simulink model "correlator_core"  (Simulink 7.1)
settings: Solver=ode45  StartTime=0.0  StopTime=10000  RelTol=1e-3
libraries: xbsIndex_r4 x658, cfa_library x168, casper_library_delays x4, casper_library_misc x2
(part 1 of 9)
settings Model: Creator=Administrator  LastModifiedBy=Rurik A Primiani

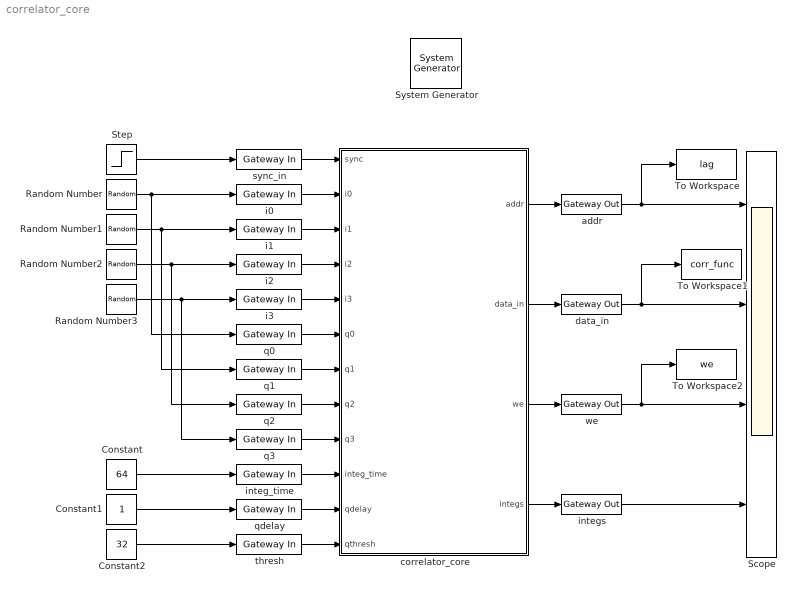
== system correlator_core ==
  " System Generator" : xbsIndex_r4/ System Generator  Tag=genX  SystemSampleTime=-1  xilinxfamily=virtex2p  part=xc2vp50  speed=-7  package=ff1152  synthesis_tool=XST  clock_wrapper=Clock Enables  directory=./correlator_core  testbench=off  simulink_period=1  sysclk_period=100  dcm_input_clock_period=100  incr_netlist=off  trim_vbits=Everywhere in SubSystem  dbl_ovrd=According to Block Masks  core_generation=According to Block Masks  run_coregen=off  deprecated_control=off  eval_field=0  block_type=sysgen
      settings: block_version=10.1.3
  Constant : Constant  Value=64  OutDataType=sfix(16)  OutScaling=2^0
  Constant1 : Constant  OutDataType=sfix(16)  OutScaling=2^0
  Constant2 : Constant  Value=32  OutDataType=sfix(16)  OutScaling=2^0
  Random Number{,1..3} (4 alike) : RandomNumber  Variance=128  Seed=ceil(1000*rand())  SampleTime=0
  Scope : Scope  NumInputPorts=4
      settings: YMin=0~-5e+006~-5~-5  YMax=32.5~5e+007~5~5
  Step : Step  Time=100  SampleTime=0
  To Workspace : ToWorkspace  VariableName=lag  SampleTime=-1  SaveFormat=Array
  To Workspace1 : ToWorkspace  VariableName=corr_func  SampleTime=-1  SaveFormat=Array
  To Workspace2 : ToWorkspace  VariableName=we  SampleTime=-1  SaveFormat=Array
  addr : xbsIndex_r4/Gateway Out  hdl_port=on  timing_constraint=None  locs_specified=off  LOCs={}  block_type=gatewayout
      settings: infoedit="Gateway out block.  Converts Xilinx fixed point inputs into ouputs of type Simulink integer, double, or fixed point.<P><P>Hardware notes:  In hardware these blocks become top level output ports or are discarded, depending on how they are configured."  block_version=10.1.3
  correlator_core : Subsystem
  data_in : xbsIndex_r4/Gateway Out  hdl_port=on  timing_constraint=None  locs_specified=off  LOCs={}  block_type=gatewayout
      settings: infoedit="Gateway out block.  Converts Xilinx fixed point inputs into ouputs of type Simulink integer, double, or fixed point.<P><P>Hardware notes:  In hardware these blocks become top level output ports or are discarded, depending on how they are configured."  block_version=10.1.3
  i{0..3} (4 alike) : xbsIndex_r4/Gateway In  arith_type="Signed  (2's comp)"  n_bits=8  bin_pt=7  quantization=Truncate  overflow=Wrap  period=1  dbl_ovrd=off  timing_constraint=None  locs_specified=off  LOCs={}  block_type=gatewayin
      settings: infoedit="Gateway in block.  Converts inputs of type Simulink integer, double and fixed point to  Xilinx fixed point type.<P><P>Hardware notes:  In hardware these blocks become top level input ports."  block_version=10.1.3
  integ_time : xbsIndex_r4/Gateway In  arith_type=Unsigned  n_bits=32  bin_pt=0  quantization=Truncate  overflow=Wrap  period=1  dbl_ovrd=off  timing_constraint=None  locs_specified=off  LOCs={}  block_type=gatewayin
      settings: infoedit="Gateway in block.  Converts inputs of type Simulink integer, double and fixed point to  Xilinx fixed point type.<P><P>Hardware notes:  In hardware these blocks become top level input ports."  block_version=10.1.3
  integs : xbsIndex_r4/Gateway Out  hdl_port=on  timing_constraint=None  locs_specified=off  LOCs={}  block_type=gatewayout
      settings: infoedit="Gateway out block.  Converts Xilinx fixed point inputs into ouputs of type Simulink integer, double, or fixed point.<P><P>Hardware notes:  In hardware these blocks become top level output ports or are discarded, depending on how they are configured."  block_version=10.1.3
  q{0..3} (4 alike) : xbsIndex_r4/Gateway In  arith_type="Signed  (2's comp)"  n_bits=8  bin_pt=7  quantization=Truncate  overflow=Wrap  period=1  dbl_ovrd=off  timing_constraint=None  locs_specified=off  LOCs={}  block_type=gatewayin
      settings: infoedit="Gateway in block.  Converts inputs of type Simulink integer, double and fixed point to  Xilinx fixed point type.<P><P>Hardware notes:  In hardware these blocks become top level input ports."  block_version=10.1.3
  qdelay : xbsIndex_r4/Gateway In  arith_type=Unsigned  n_bits=11  bin_pt=0  quantization=Truncate  overflow=Wrap  period=1  dbl_ovrd=off  timing_constraint=None  locs_specified=off  LOCs={}  block_type=gatewayin
      settings: infoedit="Gateway in block.  Converts inputs of type Simulink integer, double and fixed point to  Xilinx fixed point type.<P><P>Hardware notes:  In hardware these blocks become top level input ports."  block_version=10.1.3
  sync_in : xbsIndex_r4/Gateway In  arith_type=Boolean  n_bits=16  bin_pt=14  quantization="Round  (unbiased: +/- Inf)"  overflow=Saturate  period=1  dbl_ovrd=off  timing_constraint=None  locs_specified=off  LOCs={}  block_type=gatewayin
      settings: infoedit="Gateway in block.  Converts inputs of type Simulink integer, double and fixed point to  Xilinx fixed point type.<P><P>Hardware notes:  In hardware these blocks become top level input ports."  block_version=10.1.3
  thresh : xbsIndex_r4/Gateway In  arith_type=Unsigned  n_bits=7  bin_pt=0  quantization=Truncate  overflow=Wrap  period=1  dbl_ovrd=off  timing_constraint=None  locs_specified=off  LOCs={}  block_type=gatewayin
      settings: infoedit="Gateway in block.  Converts inputs of type Simulink integer, double and fixed point to  Xilinx fixed point type.<P><P>Hardware notes:  In hardware these blocks become top level input ports."  block_version=10.1.3
  we : xbsIndex_r4/Gateway Out  hdl_port=on  timing_constraint=None  locs_specified=off  LOCs={}  block_type=gatewayout
      settings: infoedit="Gateway out block.  Converts Xilinx fixed point inputs into ouputs of type Simulink integer, double, or fixed point.<P><P>Hardware notes:  In hardware these blocks become top level output ports or are discarded, depending on how they are configured."  block_version=10.1.3
  wires:
  sync_in/1 -> correlator_core/1(sync)
  i0/1 -> correlator_core/2(i0)
  i1/1 -> correlator_core/3(i1)
  i2/1 -> correlator_core/4(i2)
  i3/1 -> correlator_core/5(i3)
  q0/1 -> correlator_core/6(q0)
  q1/1 -> correlator_core/7(q1)
  q2/1 -> correlator_core/8(q2)
  q3/1 -> correlator_core/9(q3)
  correlator_core/1(addr) -> addr/1
  correlator_core/2(data_in) -> data_in/1
  correlator_core/3(we) -> we/1
  Random Number/1 -> i0/1, q0/1
  Random Number1/1 -> i1/1, q1/1
  Random Number2/1 -> i2/1, q2/1
  Random Number3/1 -> i3/1, q3/1
  Step/1 -> sync_in/1
  correlator_core/4(integs) -> integs/1
  integ_time/1 -> correlator_core/10(integ_time)
  Constant/1 -> integ_time/1
  addr/1 -> Scope/1, To Workspace/1
  data_in/1 -> Scope/2, To Workspace1/1
  we/1 -> Scope/3, To Workspace2/1
  integs/1 -> Scope/4
  Constant1/1 -> qdelay/1
  qdelay/1 -> correlator_core/11(qdelay)
  thresh/1 -> correlator_core/12(qthresh)
  Constant2/1 -> thresh/1

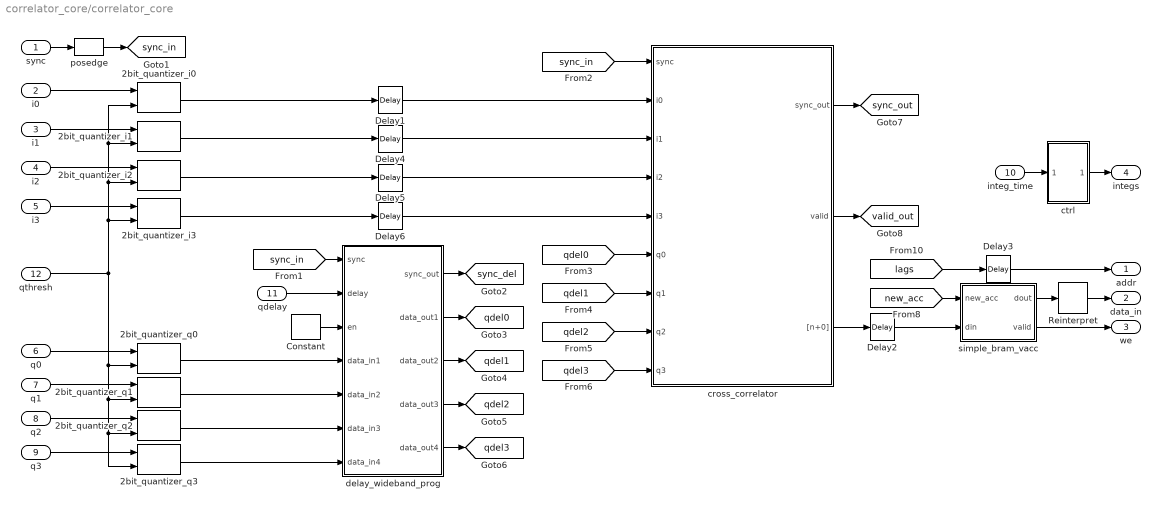
== system correlator_core/correlator_core ==
  sync : Inport
  i0 : Inport  Port=2
  i1 : Inport  Port=3
  i2 : Inport  Port=4
  i3 : Inport  Port=5
  q0 : Inport  Port=6
  q1 : Inport  Port=7
  q2 : Inport  Port=8
  q3 : Inport  Port=9
  integ_time : Inport  Port=10
  qdelay : Inport  Port=11
  qthresh : Inport  Port=12
  2bit_quantizer_i{0..3} (4 alike) : cfa_library/2bit_quantizer  SystemSampleTime=-1  relational_delay=3
  2bit_quantizer_q{0..3} (4 alike) : cfa_library/2bit_quantizer  SystemSampleTime=-1  relational_delay=3
  Constant : xbsIndex_r4/Constant  arith_type=Boolean  const=1  n_bits=16  bin_pt=14  explicit_period=on  period=1  equ=P=C  opselect=C  inp2=PCIN>>17  opr=+  inp1=P  carry=CIN  dbl_ovrd=off  block_type=constant
  Delay{1,4..6} (4 alike) : xbsIndex_r4/Delay  en=off  latency=5  dbl_ovrd=off  reg_retiming=off  block_type=delay
      settings: block_version=11.4
  Delay2 : xbsIndex_r4/Delay  en=off  latency=2  dbl_ovrd=off  reg_retiming=off  block_type=delay
      settings: block_version=11.4
  Delay3 : xbsIndex_r4/Delay  en=off  latency=3  dbl_ovrd=off  reg_retiming=off  block_type=delay
      settings: block_version=11.4
  Reinterpret : xbsIndex_r4/Reinterpret  force_arith_type=off  arith_type=Unsigned  force_bin_pt=on  bin_pt=0  block_type=reinterpret
      settings: infoedit="Changes signal type without altering the binary representation.   You can changed the signal between signed and unsigned, and relocate the binary point.<P><P>Hardware notes: In hardware this block costs nothing.<P><P>Example:  Suppose the input is 6 bits wide, signed, with 2 fractional bits, and the output is forced to unsigned with 0 fractional bits.  Then an input of -2.0 (1110.00 in binary 2's complement) becomes an output of 56 (111000 in binary)."  block_version=10.1.3
  cross_correlator : Subsystem  AncestorBlock=cfa_library/cross_correlator  mask(cross_correlator){total_lags=5, n_inputs=2, use_2bit=on, input_bit_width=8, input_bin_pt=7, specify_data_type=off, output_bit_width=16, output_bin_pt=14, quantization=Truncate, overflow=Wrap, specify_mult=off, mult_spec=Behavioral, specify_add=off, add_spec=Fabric, mult_delay=3, add_delay=2, overall_delay=2, single_output=on}
      mask prompts: total_lags "Total Lags Centered at Zero: (2^?)"; n_inputs "Number of Simultaneous Inputs: (2^?)"; use_2bit "Use special 2-bit binary encoding"; input_bit_width "Input Bit Width:"; input_bin_pt "Input Binary Point:"; specify_data_type "Specify output data type"; output_bit_width "Output Bit Width:"; output_bin_pt "Output Binary Point:"; quantization "Quantization Behavior:"; overflow "Overflow Behavior"; specify_mult "Specify multiplier use (behavioural HDL if not specified)"; mult_spec "Multiplier specification:"; specify_add "Specify adder use (behavioural HDL if not specified)"; add_spec "Adder specification:"; mult_delay "Mult Latency:"; add_delay "Add Latency:"; overall_delay "Overall latency:"; single_output "Provide single output stream"
      mask help: This time-domain cross correlator accepts two real time-series and outputs the cross-correlation function for the given set of lags. The output is accumulated so that for every two input samples there is exactly one output sample.
      mask init:
      | cross_correlator_init(gcb,...
      |     'total_lags', total_lags,...
      |     'n_inputs', n_inputs,...
      |     'use_2bit', use_2bit,...
      |     'input_bit_width', input_bit_width,...
      |     'input_bin_pt', input_bin_pt,...
      |     'specify_data_type', specify_data_type,...
      |     'output_bit_width', output_bit_width,...
      |     'output_bin_pt', output_bin_pt,...
      |     'quantization', quantization,...
      |     'overflow', overflow,...
      |     'specify_mult', specify_mult,...
      |     'mult_spec', mult_spec,...
      |     'specify_add', specify_add,...
      |     'add_spec', add_spec,...
      |     'mult_delay', mult_delay,...
      |     'add_delay', add_delay,...
      |     'overall_delay', overall_delay,...
      |     'single_output', single_output);
      settings: AttributesFormatString=|
      | 32 lags, Demux: 4, Outputs: 1
      | Special 2-bit binary encoding
      |  Mult: Behavioral, Add: Fabric
      mask StyleString: edit,edit,checkbox,edit,edit,checkbox,edit,edit,popup(Truncate|Round (unbiased: +/- Inf)|Round (unbiased: Even Values)),popup(Wrap|Saturate|Flag as error),checkbox,popup(Behavioral|Core|Embedded),checkbox,popup(Fabric|DSP48),edit,edit,edit,checkbox
      mask CallbackString:
      | ||use_2bit = get_param(gcb,'use_2bit');
      | enables = get_param(gcb, 'MaskEnables');
      | if( strcmp(use_2bit,'on')),
      |     enables{4} = 'off';
      |     enables{5} = 'off';
      | else
      |     enables{4} = 'on';
      |     enables{5} = 'on';
      | end
      | set_param(gcb, 'MaskEnables', enables);
      | |||specify_data_type = get_param(gcb,'specify_data_type');
      | enables = get_param(gcb, 'MaskEnables');
      | if( strcmp(specify_data_type,'off')),
      |     enables{7} = 'off';
      |     enables{8} = 'off';
      |     enables{9} = 'off';
      |     enables{10} = 'off';
      | else
      |     enables{7} = 'on';
      |     enables{8} = 'on';
      |     enables{9} = 'on';
      |     enables{10} = 'on';
      | end
      | set_param(gcb, 'MaskEnables', enables);
      | |||||specify_mult = get_param(gcb,'specify_mult');
      | enables = get_param(gcb, 'MaskEnables');
      | if( strcmp(specify_mult,'off')),
      |     enables{12} = 'off';
      | else
      |     enables{12} = 'on';
      | end
      | set_param(gcb, 'MaskEnables', enables);
      | ||specify_add = get_param(gcb,'specify_add');
      | enables = get_param(gcb, 'MaskEnables');
      | if( strcmp(specify_add,'off')),
      |     enables{14} = 'off';
      | else
      |     enables{14} = 'on';
      | end
      | set_param(gcb, 'MaskEnables', enables);
      | |||||
      mask TabNameString: Basic,Basic,Input,Input,Input,Output,Output,Output,Output,Output,Implementation,Implementation,Implementation,Implementation,Implementation,Implementation,Implementation,Basic
  ctrl : Subsystem
      mask Display: fprintf('CTRL');
  delay_wideband_prog : Subsystem  AncestorBlock=casper_library_delays/delay_wideband_prog  mask(delay_wideband_prog){max_delay=2048, n_inputs_bits=2, bram_latency=2, bram_type=Dual Port}
      mask prompts: max_delay "Max Delay (Sample Clks)"; n_inputs_bits "Number of Simultaneous Inputs(2^?)"; bram_latency "BRAM Latency"; bram_type "Select type of BRAM"
      mask init:
      | delay_wideband_prog_init(gcb,...
      |     'max_delay',max_delay,...
      |     'n_inputs_bits',n_inputs_bits,...
      |     'bram_latency',bram_latency,...
      |     'bram_type',bram_type);
      mask StyleString: edit,edit,edit,popup(Single Port|Dual Port)
  posedge : casper_library_misc/posedge  Tag=Rising Edge Detector  SystemSampleTime=-1
  simple_bram_vacc : Subsystem  mask(simple_bram_vacc){vec_len=32, arith_type=Signed, n_bits=32, bin_pt=14, add_latency=3}
      mask prompts: vec_len "Vector length:"; arith_type "Output type:"; n_bits "Bit width (output):"; bin_pt "Binary point (output):"; add_latency "Adder latency:"
      mask help: This simple vector accumulator is based on a shift register. It outputs its previous accumulated vector after a new_acc pulse is received.
      mask init:
      | simple_bram_vacc_init(gcb, ...
      |     'vec_len', vec_len, ...
      |     'arith_type', arith_type, ...
      |     'n_bits', n_bits, ...
      |     'bin_pt', bin_pt);
      mask StyleString: edit,popup(Signed|Unsigned),edit,edit,edit
  addr : Outport
  data_in : Outport  Port=2
  we : Outport  Port=3
  integs : Outport  Port=4
  tag scope: qdel0=global, qdel1=global, qdel2=global, qdel3=global, sync_del=global, sync_in=global, sync_out=global, valid_out=global
  wires:
  Delay2/1 -> simple_bram_vacc/2(din)
  [lags] -> Delay3/1
  [new_acc] -> simple_bram_vacc/1(new_acc)
  simple_bram_vacc/1(dout) -> Reinterpret/1
  sync/1 -> posedge/1
  Delay3/1 -> addr/1
  Reinterpret/1 -> data_in/1
  simple_bram_vacc/2(valid) -> we/1
  integ_time/1 -> ctrl/1(integ_time)
  ctrl/1(integs) -> integs/1
  Constant/1 -> delay_wideband_prog/3(en)
  qdelay/1 -> delay_wideband_prog/2(delay)
  posedge/1 -> [sync_in]
  [sync_in] -> delay_wideband_prog/1(sync)
  delay_wideband_prog/1(sync_out) -> [sync_del]
  delay_wideband_prog/2(data_out1) -> [qdel0]
  delay_wideband_prog/3(data_out2) -> [qdel1]
  delay_wideband_prog/4(data_out3) -> [qdel2]
  delay_wideband_prog/5(data_out4) -> [qdel3]
  2bit_quantizer_q0/1 -> delay_wideband_prog/4(data_in1)
  2bit_quantizer_q1/1 -> delay_wideband_prog/5(data_in2)
  2bit_quantizer_q2/1 -> delay_wideband_prog/6(data_in3)
  2bit_quantizer_q3/1 -> delay_wideband_prog/7(data_in4)
  2bit_quantizer_i0/1 -> Delay1/1
  2bit_quantizer_i1/1 -> Delay4/1
  2bit_quantizer_i2/1 -> Delay5/1
  2bit_quantizer_i3/1 -> Delay6/1
  i0/1 -> 2bit_quantizer_i0/1
  i1/1 -> 2bit_quantizer_i1/1
  i2/1 -> 2bit_quantizer_i2/1
  i3/1 -> 2bit_quantizer_i3/1
  q0/1 -> 2bit_quantizer_q0/1
  q1/1 -> 2bit_quantizer_q1/1
  q2/1 -> 2bit_quantizer_q2/1
  q3/1 -> 2bit_quantizer_q3/1
  qthresh/1 -> 2bit_quantizer_i0/2, 2bit_quantizer_i1/2, 2bit_quantizer_i2/2, 2bit_quantizer_i3/2, 2bit_quantizer_q0/2, 2bit_quantizer_q1/2, 2bit_quantizer_q2/2, 2bit_quantizer_q3/2
  cross_correlator/1(sync_out) -> [sync_out]
  cross_correlator/2(valid) -> [valid_out]
  cross_correlator/3("[n+0]") -> Delay2/1
  [sync_in] -> cross_correlator/1(sync)
  Delay1/1 -> cross_correlator/2(i0)
  Delay4/1 -> cross_correlator/3(i1)
  Delay5/1 -> cross_correlator/4(i2)
  Delay6/1 -> cross_correlator/5(i3)
  [qdel0] -> cross_correlator/6(q0)
  [qdel1] -> cross_correlator/7(q1)
  [qdel2] -> cross_correlator/8(q2)
  [qdel3] -> cross_correlator/9(q3)
